simulink model "Circuit2_alexidea"  (R2020b)
settings: Solver=ode4  StartTime=0.0  StopTime=5  FixedStep=1e-4  RelTol=1e-3
values from neighbouring files (symbols this model uses):
  Be = 1300e6    (= 1300000000)    [Circuit1_load.m]    (also in Circuit2_values.m)
  Cd = 0.7    [Circuit1_load.m]    (also in Circuit2_values.m)
  Dorifice = 2e-2    (= 0.02)    [Circuit1_load.m]    (also in Circuit2_values.m = 0.004)
  Kp = (1.e-3)/(10e5)    (= 1e-09)    [Circuit1_load.m]    (also in Circuit2_values.m; Circut3_values.m)
  pref = 180e5    (= 18000000)    [Circuit1_load.m]    (also in Circuit2_values.m; Circut3_values.m = 17000000)
  rho = 860    [Circuit1_load.m]    (also in Circuit2_values.m; Circut3_values.m)
  tau = 60e-3    (= 0.06)    [Circuit1_load.m]    (also in Circuit2_values.m = 0.03)
  V = 3e-3    (= 0.003)    [Circuit1_load.m]    (also in Circuit2_values.m)
settings Model: Creator=Janne  LastModifiedBy=Alex
settings DataIOCC: ReturnWorkspaceOutputs=off
settings DebuggingCC: ArithmeticOperatorsInVariantConditions=warning
settings SFSimCC: CustomCodeUndefinedFunction=UseInterfaceOnly

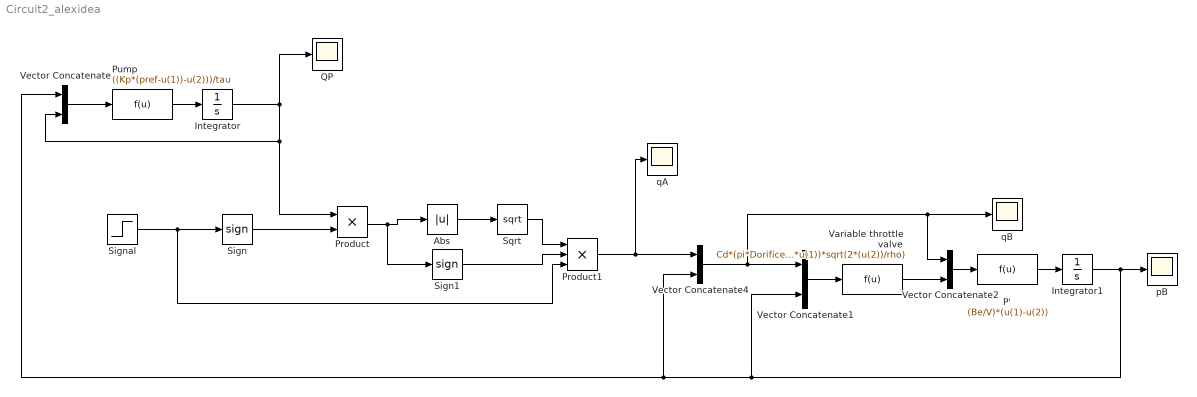
== system Circuit2_alexidea ==
  Abs : Abs
  Integrator : Integrator  LimitOutput=on  UpperSaturationLimit=1000e5  LowerSaturationLimit=0
  Integrator1 : Integrator
  P' : Fcn  Expr=(Be/V)*(u(1)-u(2))
  Product : Product
  Product1 : Product  Inputs=3
  Pump : Fcn  Expr=((Kp*(pref-u(1))-u(2)))/tau
  QP : Scope
  Sign : Signum
  Sign1 : Signum
  Signal : Step  Time=2  After=0.004  SampleTime=0
  Sqrt : Sqrt  SaturateOnIntegerOverflow=on
  Variable throttle valve : Fcn  Expr=Cd*(pi*Dorifice*u(1))*sqrt(2*(u(2))/rho)
  Vector Concatenate{,1..2,4} (4 alike) : Concatenate
  pB : Scope
  qA : Scope
  qB : Scope
  wires:
  Pump/1 -> Integrator/1
  Vector Concatenate/1 -> Pump/1
  Integrator/1 -> Product/1, Vector Concatenate/2, QP/1
  Integrator1/1 -> Vector Concatenate4/2, Vector Concatenate/1, Vector Concatenate1/2, pB/1
  Signal/1 -> Product1/3, Sign/1
  Vector Concatenate1/1 -> Variable throttle valve/1
  Variable throttle valve/1 -> Vector Concatenate2/2
  Vector Concatenate2/1 -> P'/1
  P'/1 -> Integrator1/1
  Vector Concatenate4/1 -> Vector Concatenate2/1, qB/1, Vector Concatenate1/1
  Sign/1 -> Product/2
  Abs/1 -> Sqrt/1
  Product/1 -> Sign1/1, Abs/1
  Sqrt/1 -> Product1/1
  Sign1/1 -> Product1/2
  Product1/1 -> qA/1, Vector Concatenate4/1
